simulink model "RocketPlant_harness"  (R2025b)
settings: Solver=VariableStepAuto  StartTime=0.0  StopTime=10  RelTol=1e-3
InitFcn:
  | plant_parameters;
  | fluid_constants;
  | 
  | controller_mode = controller_modes.PRESSURE;
model workspace (MAT data in the model file):
  controller_mode : controller_modes (value not decoded)
settings Model: Creator=karadeli  LastModifiedBy=Kaan Kalkandelen

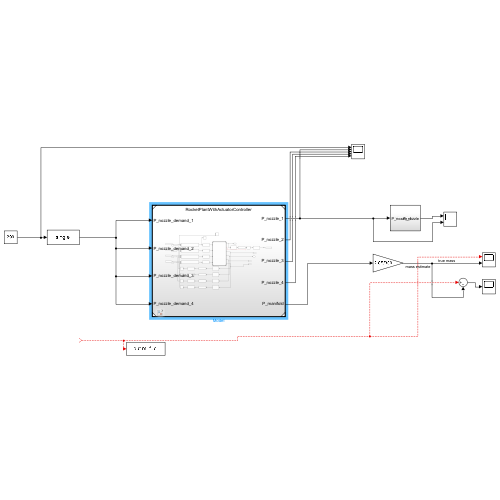
[thumbnail: Simulink's stored preview of the top-level diagram]
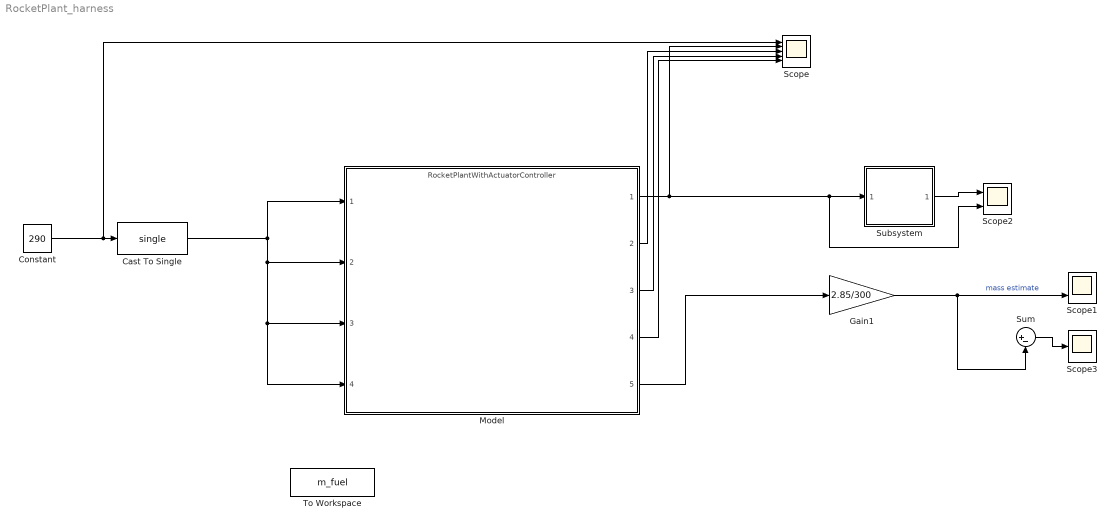
== system RocketPlant_harness ==
  Cast To Single : DataTypeConversion  OutDataTypeStr=single  SaturateOnIntegerOverflow=off  RndMeth=Floor
  Constant : Constant  Value=290
  Gain1 : Gain  Gain=2.85/300
  Model : ModelReference  ModelNameDialog=RocketPlantWithActuatorController.slx  SimulationMode=Normal  ModelReferenceVersion=1.30
  Scope : Scope  NumInputPorts=5
      settings: ActiveDisplayYMinimum=-16.249999999999996  ActiveDisplayYMaximum=146.25
  Scope1 : Scope  NumInputPorts=2
      settings: ActiveDisplayYMinimum=-0.35214846070629818  ActiveDisplayYMaximum=3.2057942734118114
  Scope2 : Scope  NumInputPorts=2
      settings: ActiveDisplayYMinimum=-243.01530735239314  ActiveDisplayYMaximum=381.79572212955406  DataLoggingVariableName=ScopeData2
  Scope3 : Scope
      settings: ActiveDisplayYMinimum=-0.07057443305678722  ActiveDisplayYMaximum=0.626703618894777  DataLoggingVariableName=ScopeData3
  Subsystem : Subsystem
  Sum : Sum  Inputs=|+-
  To Workspace : ToWorkspace  VariableName=m_fuel  SaveFormat=Timeseries  SampleTime=-1
  wires:
  Model/1 -> Scope/2, Scope2/2, Subsystem/1(P_nozzle_1)
  Model/2 -> Scope/3
  Constant/1 -> Scope/1, Cast To Single/1
  Cast To Single/1 -> Model/4, Model/3, Model/2, Model/1
  Model/3 -> Scope/4
  Model/4 -> Scope/5
  Subsystem/1(F_nozzle) -> Scope2/1
  Model/5 -> Gain1/1
  ? -> Scope1/1, Sum/1, To Workspace/1  "true mass"
  Gain1/1 -> Sum/2, Scope1/2  "mass estimate"
  Sum/1 -> Scope3/1

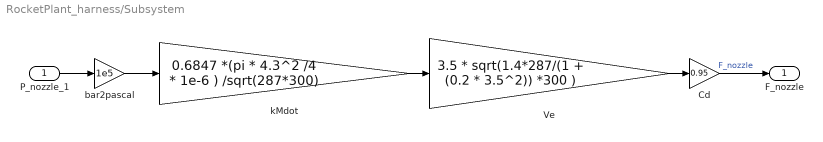
== system RocketPlant_harness/Subsystem ==
  P_nozzle_1 : Inport  Unit=bar
  Cd : Gain  Gain=0.95
  Ve : Gain  Gain=3.5 * sqrt(1.4*287/(1 + (0.2 * 3.5^2)) *300 )
  bar2pascal : Gain  Gain=1e5
  kMdot : Gain  Gain=0.6847 *(pi * 4.3^2 /4 * 1e-6 ) /sqrt(287*300)
  F_nozzle : Outport  Unit=N
  wires:
  Cd/1 -> F_nozzle/1  "F_nozzle"
  P_nozzle_1/1 -> bar2pascal/1
  Ve/1 -> Cd/1
  kMdot/1 -> Ve/1
  bar2pascal/1 -> kMdot/1
